simulink model "obserwator"  (R2022a)
settings: Solver=VariableStepAuto  StartTime=0.0  StopTime=10.0  RelTol=1e-3
values from neighbouring files (symbols this model uses):
  L1 = -(14149*so)/30 - (781*so^2)/15 - (347*so^3)/180 - 130493/90    (= 415.827777778)    [dane.m]
  L2 = (77*so^3)/360 + (347*so^2)/60 + (781*so)/15 + 14149/90    (= -44.4138888889)    [dane.m]
  L3 = -(347*so)/60 - (77*so^2)/120 - (17*so^3)/720 - 781/45    (= 4.70694444444)    [dane.m]
settings Model: Creator=danie  LastModifiedBy=danie

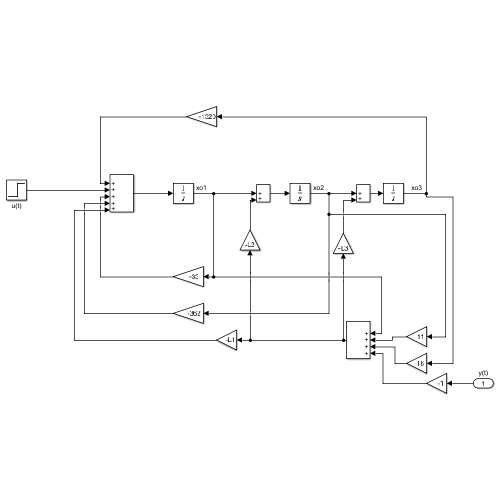
[thumbnail: Simulink's stored preview of the top-level diagram]
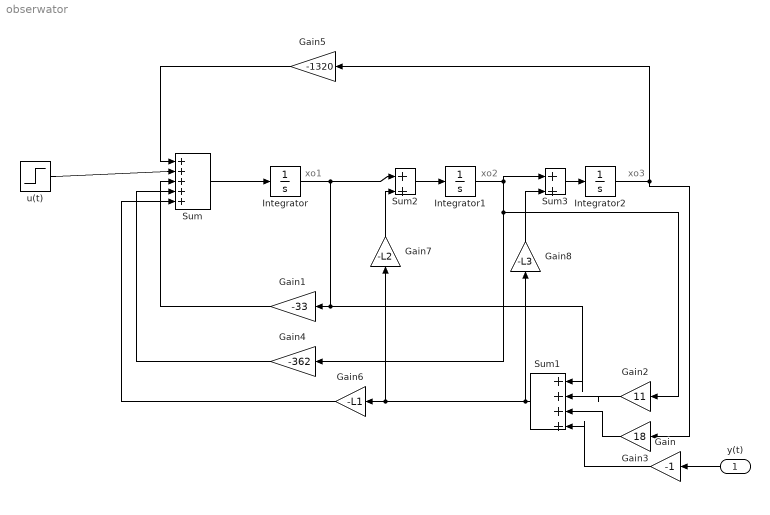
== system obserwator ==
  note: xo1
  note: xo2
  note: xo3
  y(t) : Inport
  Gain : Gain  Gain=-1
  Gain1 : Gain  Gain=-33
  Gain2 : Gain  Gain=11
  Gain3 : Gain  Gain=18
  Gain4 : Gain  Gain=-362
  Gain5 : Gain  Gain=-1320
  Gain6 : Gain  Gain=-L1
  Gain7 : Gain  Gain=-L2
  Gain8 : Gain  Gain=-L3
  Integrator : Integrator
  Integrator1 : Integrator
  Integrator2 : Integrator
  Sum : Sum  Inputs=|+++++
  Sum1 : Sum  Inputs=|++++
  Sum2 : Sum  Inputs=|++
  Sum3 : Sum  Inputs=|++
  u(t) : Step  SampleTime=0
  wires:
  Sum/1 -> Integrator/1
  Integrator/1 -> Sum1/1, Gain1/1, Sum2/1
  Integrator1/1 -> Gain2/1, Gain4/1, Sum3/1
  Gain2/1 -> Sum1/2
  Integrator2/1 -> Gain3/1, Gain5/1
  Gain3/1 -> Sum1/3
  Sum1/1 -> Gain7/1, Gain6/1, Gain8/1
  Gain5/1 -> Sum/1
  u(t)/1 -> Sum/2
  Gain1/1 -> Sum/3
  Gain4/1 -> Sum/4
  Gain6/1 -> Sum/5
  y(t)/1 -> Gain/1
  Gain/1 -> Sum1/4
  Sum2/1 -> Integrator1/1
  Sum3/1 -> Integrator2/1
  Gain8/1 -> Sum3/2
  Gain7/1 -> Sum2/2
